simulink model "RigidCar_20230613_Plots"  (R2022b)
settings: Solver=ode1  StartTime=0.0  StopTime=35  FixedStep=0.0001  RelTol=1e-3
model workspace (MAT data in the model file):
  Mu = [0.1; 0.1; 0; 0]
  x_init = [5; 0; 0]
libraries: simulink_extras x1
settings Model: Creator=giuli  LastModifiedBy=simob

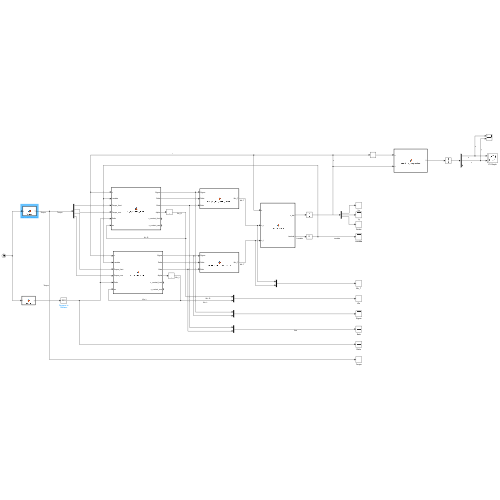
[thumbnail: Simulink's stored preview of the top-level diagram]
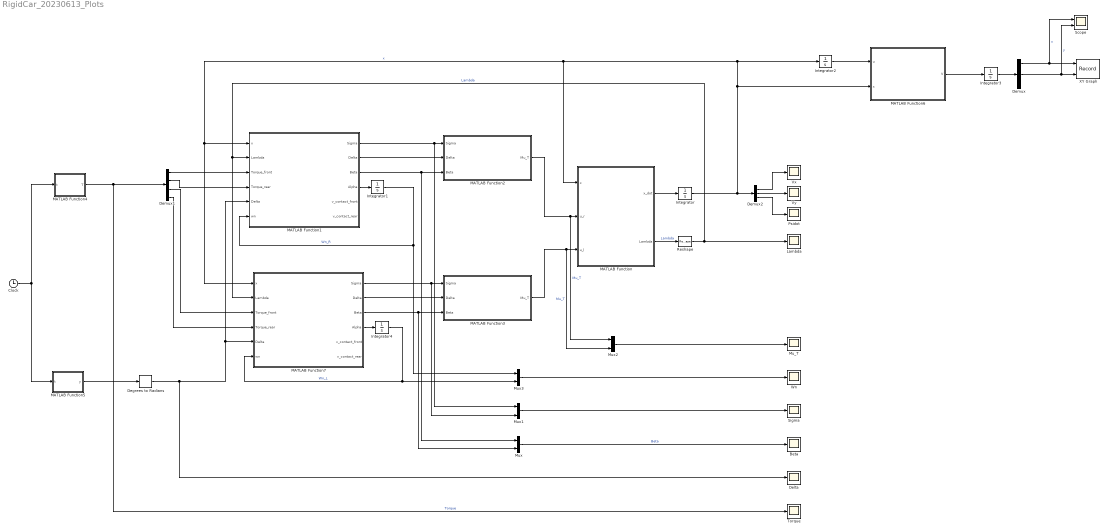
== system RigidCar_20230613_Plots ==
  Beta : Scope
  Clock : Clock
  Degrees to Radians : simulink_extras/Transformations/Degrees to Radians
  Delta : Scope
  Demux : Demux  Outputs=3
  Demux1 : Demux
  Demux2 : Demux  Outputs=3
  Integrator : Integrator  InitialCondition=x_init
  Integrator1 : Integrator  InitialCondition=[x_init(1)/0.25; x_init(1)/0.25]
  Integrator2 : Integrator  InitialCondition=[0; 0; 0]
  Integrator3 : Integrator  InitialCondition=[0; 0; 0]
  Integrator4 : Integrator  InitialCondition=[x_init(1)/0.25; x_init(1)/0.25]
  Lambda : Scope
  MATLAB Function : MATLAB Function  TreatAsAtomicUnit=on
  MATLAB Function1 : MATLAB Function  TreatAsAtomicUnit=on
  MATLAB Function2 : MATLAB Function  TreatAsAtomicUnit=on
  MATLAB Function3 : MATLAB Function  TreatAsAtomicUnit=on
  MATLAB Function4 : MATLAB Function  TreatAsAtomicUnit=on
  MATLAB Function5 : MATLAB Function  TreatAsAtomicUnit=on
  MATLAB Function6 : MATLAB Function  TreatAsAtomicUnit=on
  MATLAB Function7 : MATLAB Function  TreatAsAtomicUnit=on
  Mu_T : Scope
  Mux{,1..3} (4 alike) : Mux  Inputs=2
  Psidot : Scope
  Reshape : Reshape  OutputDimensionality=Customize  OutputDimensions=[4,1]
  Scope : Scope  NumInputPorts=2
  Sigma : Scope
  Torque : Scope
  Vx : Scope
  Vy : Scope
  Wn : Scope
  XY Graph : Record  FileSettingsInternal="{\"entries\":[{\"content\":{\"excelSettings\":{\"content\":{},\"type\":\"Streamout.ExcelSettings\"}},\"type\":\"Streamout.FileSettingStorage\",\"uuid\":\"046155c9-5b4d-406d-a542-4821e8795aa4\"}],\"packageUris\":[\"http://schema.mathworks.com/mf0/streamout_blocks/R2020a\"],\"version\":\"1.0\"}"  Layout=[1 1]  SignalsInternal="{\"entries\":[{\"content\":{\"signals\":[{\"content\":{\"blockPath\":[\"RigidCar_20230616/XY Graph\"],\"channel\":[],\"dimensions\":[1,1],\"domain\":\"RigidCar_20230616/XY Graph\",\"lineColor\":\"#a2142f\",\"plots\":[1],\"port\":1,\"sid\":[\"\"],\"signalID\":24208,\"signalName\":\"x\"},\"type\":\"RecordBlkView.Signal\",\"uuid\":\"78936cc0-01b6-44d5-a461-2239488a3985\"},{\"content\":{\"blockPath\":[\"RigidCar_20230616/XY Graph\"],\"channel\":[],\"dimensions\":[1,1],\"domain\":\"RigidCar_20230616/XY Graph\",\"lineColor\":\"#139fff\",\"plots\":[1],\"port\":2,\"sid\":[\"\"],\"signalID\":24212,\"signalName\":\"y\"},\"type\":\"RecordBlkView.Signal\",\"uuid\":\"a4f5c4ac-768a-465c-bd6f-86ef2aa16df8\"}]},\"type\":\"RecordBlkView.InputSignals\",\"uuid\":\"fded4382-bc6b-4d76-8cf1-91bfd3eec9ad\"}],\"packageUris\":[\"http://schema.mathworks.com/mf0/streamout_blocks/R2020a\"],\"version\":\"1.0\"}"  VisualizationBindings="{\"xyplotplugin\":{\"info\":[{\"series\":[{\"bindingParametersList\":[{\"parameter\":\"X-Axis\",\"signalID\":24208,\"signalName\":\"x\"},{\"parameter\":\"Y-Axis\",\"signalID\":24212,\"signalName\":\"y\"}],\"seriesID\":4769}],\"subplotID\":1}]}}"  CompatibilityTag=XY
  wires:
  MATLAB Function/1(x_dot) -> Integrator/1
  Integrator/1 -> Demux2/1, MATLAB Function6/2(x), Integrator2/1, MATLAB Function1/1(x), MATLAB Function7/1(x), MATLAB Function/1(x)  "x"
  MATLAB Function/2(Lambda) -> Reshape/1  "Lambda"
  MATLAB Function2/1(Mu_T) -> Mux2/1, MATLAB Function/2(u_r)  "Mu_T"
  MATLAB Function1/1(Sigma) -> MATLAB Function2/1(Sigma), Mux1/1
  MATLAB Function1/4(Alpha) -> Integrator1/1
  Integrator1/1 -> MATLAB Function1/6(wn), Mux3/1  "Wn_R"
  MATLAB Function1/2(Delta) -> MATLAB Function2/2(Delta)
  MATLAB Function1/3(Beta) -> MATLAB Function2/3(Beta), Mux/1
  Degrees to Radians/1 -> MATLAB Function1/5("Delta "), MATLAB Function7/5("Delta "), Delta/1
  MATLAB Function5/1(y) -> Degrees to Radians/1
  Clock/1 -> MATLAB Function4/1(t), MATLAB Function5/1(t)
  Integrator2/1 -> MATLAB Function6/1(u)
  MATLAB Function6/1(V) -> Integrator3/1
  Integrator3/1 -> Demux/1
  Demux/1 -> Scope/1, XY Graph/1  "x"
  Demux/2 -> Scope/2, XY Graph/2  "y"
  Reshape/1 -> MATLAB Function1/2(Lambda), MATLAB Function7/2(Lambda), Lambda/1  "Lambda"
  MATLAB Function7/4(Alpha) -> Integrator4/1
  Integrator4/1 -> Mux3/2, MATLAB Function7/6(wn)  "Wn_L"
  MATLAB Function7/1(Sigma) -> Mux1/2, MATLAB Function3/1(Sigma)
  MATLAB Function7/2(Delta) -> MATLAB Function3/2(Delta)
  MATLAB Function7/3(Beta) -> MATLAB Function3/3(Beta), Mux/2
  MATLAB Function3/1(Mu_T) -> Mux2/2, MATLAB Function/3(u_l)  "Mu_T"
  MATLAB Function4/1(T) -> Torque/1, Demux1/1  "Torque"
  Demux1/1 -> MATLAB Function1/3(Torque_front)
  Demux1/2 -> MATLAB Function1/4(Torque_rear)
  Demux1/3 -> MATLAB Function7/3(Torque_front)
  Demux1/4 -> MATLAB Function7/4(Torque_rear)
  Mux/1 -> Beta/1  "Beta"
  Mux1/1 -> Sigma/1
  Mux2/1 -> Mu_T/1
  Mux3/1 -> Wn/1
  Demux2/2 -> Vy/1
  Demux2/3 -> Psidot/1
  Demux2/1 -> Vx/1

== matlab function RigidCar_20230613_Plots/MATLAB Function1 ==
  data: Sigma output; Delta output; Beta output; x input; Lambda input; Torque_front input; Torque_rear input; Delta input; Alpha output; wn input; v_contact_front output; v_contact_rear output
function [Sigma, Delta, Beta, Alpha, v_contact_front, v_contact_rear]  = tire_dynamics_RIGHT(x, Lambda, Torque_front, Torque_rear, Delta, wn)
%Alpha = [wn_front_dot, wn_rear_dot]

%%%
a = 1.48;
b = 1.08;

bfx = 18.22;
cfx = 1.37;
dfx = 1.48;
efx = -0.46;
r1fx = 13.476;
r2fx = 11.354;

brx = 18.22;
crx = 1.37;
drx = 1.48;
erx = -0.46;
r1rx = 13.476;
r2rx = 11.354;

cxbeta = 1.1231;

tF = 0.76;
tR = 0.79;
%%%

wheel_radius = 0.25; %m
wheel_mass = 15; %kg
wheel_Inertia = 0.5*wheel_mass*(wheel_radius^2); %cylinder inertia

torque_front = Torque_front;
torque_rear = Torque_rear;

wn_front = wn(1);
wn_rear = wn(2);

Vx = x(1);
Vy = x(2);
psi_dot = x(3);

%body frame
    psi_dot_skew = [0 -psi_dot 0; psi_dot 0 0; 0 0 0];
    v_contact_front = [Vx; Vy; 0] + psi_dot_skew*[a+b; tF; 0];
    v_contact_rear = [Vx; Vy; 0]+ psi_dot_skew*[0; tR; 0];


%beta computation    
    beta_front = Delta - atan2(v_contact_front(2), v_contact_front(1));
    beta_rear = -atan2(v_contact_rear(2), v_contact_rear(1));
    Beta = [beta_front; beta_rear];

%wheel frame
    rotation_matrix = [cos(Delta) sin(Delta) 0; -sin(Delta) cos(Delta) 0; 0 0 1];
    v_contact_front = rotation_matrix*v_contact_front;
    % v_contact_rear is already fine

%sigma computation
    sigma_front = (wheel_radius*wn_front - v_contact_front(1))/v_contact_front(1);
    sigma_rear = (wheel_radius*wn_rear - v_contact_rear(1))/v_contact_rear(1);
    Sigma = [sigma_front; sigma_rear];

    fz_front = Lambda(1);
    fz_rear = Lambda(3);
    
    
    %angular velocities
    Mu_front = dfx*sin(cfx*atan(bfx*sigma_front-efx*(bfx*sigma_front-atan(bfx*sigma_front))))*cos(cxbeta*atan(beta_front*r1fx/(1+(r2fx*sigma_front)^2)));%in wheel frame
    Mu_rear = drx*sin(crx*atan(brx*sigma_rear-erx*(brx*sigma_rear-atan(brx*sigma_rear))))*cos(cxbeta*atan(beta_rear*r1rx/(1+(r2rx*sigma_rear)^2)));%in wheel frame
    Fx_front = -fz_front*Mu_front;
    Fx_rear = -fz_rear*Mu_rear;

    alpha_front = (torque_front - wheel_radius*Fx_front)/wheel_Inertia;
    alpha_rear = (torque_rear - wheel_radius*Fx_rear)/wheel_Inertia;
    Alpha = [alpha_front; alpha_rear];

    Mu = [Mu_front; Mu_rear];

== matlab function RigidCar_20230613_Plots/MATLAB Function ==
  data: x input; u_r input; x_dot output; Lambda output; u_l input
function [x_dot, Lambda] = car_dynamics(x, u_r, u_l)
m = 1528.68;
a = 1.48;
b = 1.08;
h = 0.43;
g = 9.81;
Izz = 6022.36;
Ixz = -1.91;
d = 0.0014; % Our hypotesys %
tf = 0.76;
tr = 0.79;
c_fr = 1;
c_fl = 1;
c_rr = 1;
c_rl = 1;


Vx = x(1);
Vy = x(2);
Psi_dot = x(3);
    
Mu_frx = u_r(1);
Mu_rrx = u_r(2);

Mu_fry = u_r(3);
Mu_rry = u_r(4);
        
Mu_flx = u_l(1);
Mu_rlx = u_l(2);

Mu_fly = u_l(3);
Mu_rly = u_l(4);

M = [m 0 -m*d Mu_frx Mu_flx Mu_rrx Mu_rlx;
    0 m m*b Mu_fry Mu_fly Mu_rry Mu_rly;
    -m*d m*b (Izz+m*(b^2+d^2)) ((a+b)*Mu_fry - tf*Mu_frx) ((a+b)*Mu_fly + tf*Mu_flx) (-tr*Mu_rrx) (tr*Mu_rlx);
    0 0 0 -1 -1 -1 -1;
    0 m*h (Ixz + m*b*h) -tf tf -tr tr;
    -m*h 0 (m*h*d) (a+b) (a+b) 0 0;
    0 0 0 (-c_fr*tr) (c_fl*tr) (c_rr*tf) (-c_rl*tf)];

K = [-m*Psi_dot*(Vy + b*Psi_dot);
    m*Psi_dot*(Vx - d*Psi_dot);
    m*Psi_dot*(d*Vy + b*Vx);
    -m*g;
    (m*h*Psi_dot*(Vx - d*Psi_dot)) - m*g*d;
    (m*h*Vy*Psi_dot+(Ixz +m*b*h)*(Psi_dot^2)) + m*g*b;
    0];

out = -inv(M)*K;

x_dot = out(1:3); %Vx_dot, Vy_dot, psi_doubledot
Lambda = out(4:7); %Fz_fr, Fz_fl, Fz_rr, Fz_rl

== matlab function RigidCar_20230613_Plots/MATLAB Function2 ==
  data: Sigma input; Mu_T output; Delta input; Beta input
function Mu_T = Pacejka_tire_model_RIGHT(Sigma, Delta, Beta)
%%%
bfx = 18.22;
cfx = 1.37;
dfx = 1.48;
efx = -0.46;
r1fx = 13.476;
r2fx = 11.354;

brx = 18.22;
crx = 1.37;
drx = 1.48;
erx = -0.46;
r1rx = 13.476;
r2rx = 11.354;

bfy = 17.8;
cfy = 1.25;
dfy = 1.22;
efy = 0.02;
r1fy = 7.7856;
r2fy = 8.1697;

bry = 17.8;
cry = 1.25;
dry = 1.22;
ery = 0.02;
r1ry = 7.7856;
r2ry = 8.1697;

cxbeta = 1.1231;
cysigma = 1.0533;
%%%

%%%
beta_front = Beta(1);
beta_rear = Beta(2);

sigma_front = Sigma(1);
sigma_rear = Sigma(2);
%%%

MuFx = F0_fnc(sigma_front, bfx, cfx, dfx, efx) * Gx_fnc(sigma_front, beta_front, cxbeta, r1fx, r2fx);
MuRx = F0_fnc(sigma_rear, brx, crx, drx, erx) * Gx_fnc(sigma_rear, beta_rear, cxbeta, r1rx, r2rx);
MuFy = F0_fnc(beta_front, bfy, cfy, dfy, efy) * Gy_fnc(sigma_front, beta_front, cysigma, r1fy, r2fy);
MuRy = F0_fnc(beta_rear, bry, cry, dry, ery) * Gy_fnc(sigma_rear, beta_rear, cysigma, r1ry, r2ry);

MuFx_T = MuFx*cos(Delta) - MuFy*sin(Delta);
MuRx_T = MuRx;
MuFy_T = MuFx*sin(Delta) + MuFy*cos(Delta);
MuRy_T = MuRy;

Mu_T = [MuFx_T MuRx_T MuFy_T MuRy_T];
end

function Gy = Gy_fnc(Sigma, Beta, cysigma, r1, r2) 
    Gy = cos(cysigma*atan(Sigma*r1/(1+(r2*Beta)^2)));
end

function F0 = F0_fnc(x, b, c, d, e)
    F0 = d*sin(c*atan(b*x-e*(b*x-atan(b*x))));
end

function Gx = Gx_fnc(Sigma, Beta, cxbeta, r1, r2) 
    Gx = cos(cxbeta*atan(Beta*r1/(1+(r2*Sigma)^2)));
end

== matlab function RigidCar_20230613_Plots/MATLAB Function3 ==
  data: Sigma input; Mu_T output; Delta input; Beta input
function Mu_T = Pacejka_tire_model_LEFT(Sigma, Delta, Beta)
%%%
bfx = 18.22;
cfx = 1.37;
dfx = 1.48;
efx = -0.46;
r1fx = 13.476;
r2fx = 11.354;

brx = 18.22;
crx = 1.37;
drx = 1.48;
erx = -0.46;
r1rx = 13.476;
r2rx = 11.354;

bfy = 17.8;
cfy = 1.25;
dfy = 1.22;
efy = 0.02;
r1fy = 7.7856;
r2fy = 8.1697;

bry = 17.8;
cry = 1.25;
dry = 1.22;
ery = 0.02;
r1ry = 7.7856;
r2ry = 8.1697;

cxbeta = 1.1231;
cysigma = 1.0533;
%%%

%%%
beta_front = Beta(1);
beta_rear = Beta(2);

sigma_front = Sigma(1);
sigma_rear = Sigma(2);
%%%

MuFx = F0_fnc(sigma_front, bfx, cfx, dfx, efx) * Gx_fnc(sigma_front, beta_front, cxbeta, r1fx, r2fx);
MuRx = F0_fnc(sigma_rear, brx, crx, drx, erx) * Gx_fnc(sigma_rear, beta_rear, cxbeta, r1rx, r2rx);
MuFy = F0_fnc(beta_front, bfy, cfy, dfy, efy) * Gy_fnc(sigma_front, beta_front, cysigma, r1fy, r2fy);
MuRy = F0_fnc(beta_rear, bry, cry, dry, ery) * Gy_fnc(sigma_rear, beta_rear, cysigma, r1ry, r2ry);

MuFx_T = MuFx*cos(Delta) - MuFy*sin(Delta);
MuRx_T = MuRx;
MuFy_T = MuFx*sin(Delta) + MuFy*cos(Delta);
MuRy_T = MuRy;

Mu_T = [MuFx_T MuRx_T MuFy_T MuRy_T];
end

function Gy = Gy_fnc(Sigma, Beta, cysigma, r1, r2) 
    Gy = cos(cysigma*atan(Sigma*r1/(1+(r2*Beta)^2)));
end

function F0 = F0_fnc(x, b, c, d, e)
    F0 = d*sin(c*atan(b*x-e*(b*x-atan(b*x))));
end

function Gx = Gx_fnc(Sigma, Beta, cxbeta, r1, r2) 
    Gx = cos(cxbeta*atan(Beta*r1/(1+(r2*Sigma)^2)));
end

== matlab function RigidCar_20230613_Plots/MATLAB Function4 ==
  data: t input; T output
function T = Torque(t)
% 
% if t > 10
%      y = -100;
% else
%      y = 0;
% end

%y=250*(1/(1+exp(-0.4*(t-15))));
% if t > 10
%      y=-250*(1/(1+exp(-0.4*(t-15))));
% else
%      y=250*(1/(1+exp(-0.4*(t-15))));
% end
%y = -30*(1/(1+exp(-0.05*(t-80))));
% % y = 1400;
% y = 500*exp(-(t-5)^2/100);

% Tf_R =0;
% Tr_R = 500*exp(-(t-5)^2/100);
% Tf_L = 0;
% Tr_L = 500*exp(-(t-5)^2/100);

% if t > 5
%     y = 15*(t-5);
% 
% else
%     y = 0;
% end
% 
% 
% 
y = 150;
% 
Tf_R = y;
Tr_R = y;
Tf_L = y;
Tr_L = y;


T = [Tf_R, Tr_R, Tf_L, Tr_L];

== matlab function RigidCar_20230613_Plots/MATLAB Function5 ==
  data: t input; y output
function y = Delta(t)
%y = 3*(1/(1+exp(-0.05*(t-100))));
% if t>50
%     y=-10;
% else
%     y=0;
% end
% y = 2-2*exp(-2*t);

if t > 10
    y = 3;
else
    y = 0.3*t;
end

% y = 0;

% end

== matlab function RigidCar_20230613_Plots/MATLAB Function6 ==
  data: u input; x input; V output
function V = trajectory_computation(u,x)
psi = u(3);
Vx = x(1);
Vy = x(2);

%body frame
Vx_vect = [Vx; 0; 0];
Vy_vect = [0; Vy; 0];

%global frame
rotation_matrix = [cos(psi) sin(psi) 0; sin(psi) -cos(psi) 0; 0 0 1];
Vx_vect = rotation_matrix*Vx_vect;
Vy_vect = rotation_matrix*Vy_vect;
V = Vx_vect + Vy_vect;

== matlab function RigidCar_20230613_Plots/MATLAB Function7 ==
  data: Sigma output; Delta output; Beta output; x input; Lambda input; Torque_front input; Torque_rear input; Delta input; Alpha output; wn input; v_contact_front output; v_contact_rear output
function [Sigma, Delta, Beta, Alpha, v_contact_front, v_contact_rear]  = tire_dynamics_LEFT(x, Lambda, Torque_front, Torque_rear, Delta, wn)
%Alpha = [wn_front_dot, wn_rear_dot]

%%%
a = 1.48;
b = 1.08;

bfx = 18.22;
cfx = 1.37;
dfx = 1.48;
efx = -0.46;
r1fx = 13.476;
r2fx = 11.354;

brx = 18.22;
crx = 1.37;
drx = 1.48;
erx = -0.46;
r1rx = 13.476;
r2rx = 11.354;

cxbeta = 1.1231;

tF = 0.76;
tR = 0.79;
%%%

wheel_radius = 0.25; %m
wheel_mass = 15; %kg
wheel_Inertia = 0.5*wheel_mass*(wheel_radius^2); %cylinder inertia

torque_front = Torque_front;
torque_rear = Torque_rear;

wn_front = wn(1);
wn_rear = wn(2);

Vx = x(1);
Vy = x(2);
psi_dot = x(3);

%body frame
    psi_dot_skew = [0 -psi_dot 0; psi_dot 0 0; 0 0 0];
    v_contact_front = [Vx; Vy; 0] + psi_dot_skew*[a+b; -tF; 0];
    v_contact_rear = [Vx; Vy; 0]+ psi_dot_skew*[0; -tR; 0];
    
%beta computation    
    beta_front = Delta - atan2(v_contact_front(2), v_contact_front(1));
    beta_rear = -atan2(v_contact_rear(2), v_contact_rear(1));
    Beta = [beta_front; beta_rear];

%wheel frame
    rotation_matrix = [cos(Delta) sin(Delta) 0; -sin(Delta) cos(Delta) 0; 0 0 1];
    v_contact_front = rotation_matrix*v_contact_front;
    % v_contact_rear is already fine

%sigma computation    
    sigma_front = (wheel_radius*wn_front - v_contact_front(1))/v_contact_front(1);
    sigma_rear = (wheel_radius*wn_rear - v_contact_rear(1))/v_contact_rear(1);
    Sigma = [sigma_front; sigma_rear];

    fz_front = Lambda(2);
    fz_rear = Lambda(4);
    
    
    %angular velocities
    Mu_front = dfx*sin(cfx*atan(bfx*sigma_front-efx*(bfx*sigma_front-atan(bfx*sigma_front))))*cos(cxbeta*atan(beta_front*r1fx/(1+(r2fx*sigma_front)^2)));%in wheel frame
    Mu_rear = drx*sin(crx*atan(brx*sigma_rear-erx*(brx*sigma_rear-atan(brx*sigma_rear))))*cos(cxbeta*atan(beta_rear*r1rx/(1+(r2rx*sigma_rear)^2)));%in wheel frame
    Fx_front = -fz_front*Mu_front;
    Fx_rear = -fz_rear*Mu_rear;

    alpha_front = (torque_front - wheel_radius*Fx_front)/wheel_Inertia;
    alpha_rear = (torque_rear - wheel_radius*Fx_rear)/wheel_Inertia;
    Alpha = [alpha_front; alpha_rear];

    Mu = [Mu_front; Mu_rear];
